simulink model "pierwszy"  (R2019a)
settings: Solver=FixedStepAuto  StartTime=0.0  StopTime=20  FixedStep=0.1  MinStep=0.1  RelTol=1e-3
settings Model: Creator=ASUS_PEPE  LastModifiedBy=ASUS_PEPE

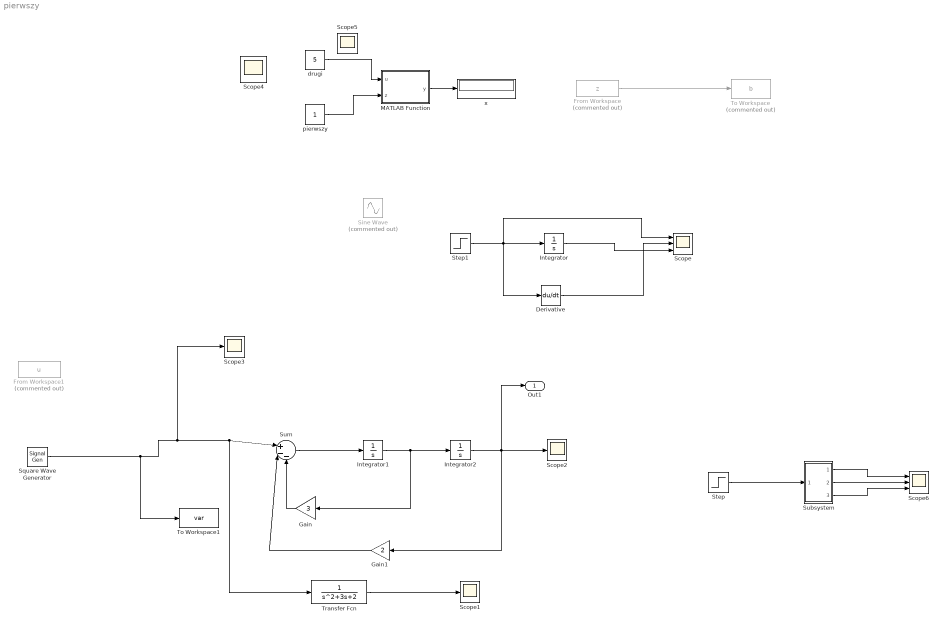
== system pierwszy ==
  Derivative : Derivative
  From Workspace : FromWorkspace  Commented=on  VariableName=z  SampleTime=0
  From Workspace1 : FromWorkspace  Commented=on  VariableName=u  SampleTime=0
  Gain : Gain  Gain=3
  Gain1 : Gain  Gain=2
  Integrator : Integrator
  Integrator1 : Integrator
  Integrator2 : Integrator
  MATLAB Function : MATLAB Function  TreatAsAtomicUnit=on
  Scope : Scope  NumInputPorts=3
  Scope{1..5} (5 alike) : Scope
  Scope6 : Scope  NumInputPorts=3
  Sine Wave : Sin  Commented=on  SampleTime=0
  Square Wave Generator : SignalGenerator  WaveForm=square  Units=rad/sec
  Step : Step  SampleTime=0
  Step1 : Step  Time=5  SampleTime=0
  Subsystem : Subsystem  mask{k1=100, k2=10, k3=55}
  Sum : Sum  Inputs=|+--
  To Workspace : ToWorkspace  Commented=on  VariableName=b  SaveFormat=Timeseries  SampleTime=-1
  To Workspace1 : ToWorkspace  VariableName=var  SampleTime=-1
  Transfer Fcn : TransferFcn  Denominator=[1 3 2]
  drugi : Constant  Value=5
  pierwszy : Constant
  x : Display
  Out1 : Outport  SignalName=x
  wires:
  Integrator/1 -> Scope/3
  Derivative/1 -> Scope/2
  Step1/1 -> Scope/1, Derivative/1, Integrator/1
  pierwszy/1 -> MATLAB Function/2(z)
  MATLAB Function/1(y) -> x/1
  drugi/1 -> MATLAB Function/1(u)
  From Workspace/1 -> To Workspace/1
  Integrator1/1 -> Gain/1, Integrator2/1
  Sum/1 -> Integrator1/1
  Transfer Fcn/1 -> Scope1/1
  Gain/1 -> Sum/3
  Gain1/1 -> Sum/2
  Integrator2/1 -> Out1/1, Gain1/1, Scope2/1
  Step/1 -> Subsystem/1(In1)
  Subsystem/1(Out1) -> Scope6/1
  Subsystem/2(Out2) -> Scope6/2
  Subsystem/3(Out3) -> Scope6/3
  Square Wave Generator/1 -> To Workspace1/1, Scope3/1, Transfer Fcn/1, Sum/1

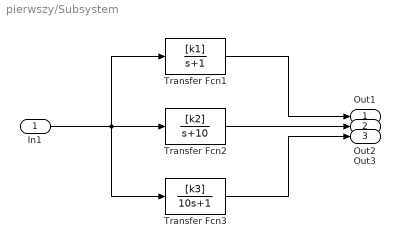
== system pierwszy/Subsystem ==
  In1 : Inport
  Transfer Fcn1 : TransferFcn  Numerator=[k1]  Denominator=[1 1]
  Transfer Fcn2 : TransferFcn  Numerator=[k2]  Denominator=[1 10]
  Transfer Fcn3 : TransferFcn  Numerator=[k3]  Denominator=[10 1]
  Out1 : Outport
  Out2 : Outport  Port=2
  Out3 : Outport  Port=3
  wires:
  Transfer Fcn1/1 -> Out1/1
  In1/1 -> Transfer Fcn3/1, Transfer Fcn1/1, Transfer Fcn2/1
  Transfer Fcn3/1 -> Out3/1
  Transfer Fcn2/1 -> Out2/1

== matlab function pierwszy/MATLAB Function ==
  data: u input; y output; z input
function y = fcn(u,z)

y = u+z;
